simulink library "Px4Library"  (R2015b)
settings: Solver=VariableStepAuto  StartTime=0.0  StopTime=10.0  RelTol=1e-3
undefined symbols (not defined in the file): armed, ctrl_state, INIT_PARAM_VECTOR, mpc_att_sp, mpc_ctrl_state, mpc_manual, mpc_pos_sp_triplet, mpc_vehicle_land_detected, mpc_vehicle_status, v_att_sp, v_control_mode
libraries: simulink x4
(part 2 of 7)

== matlab function Px4Library/mc_att_control/mc_att_control_main ==
  data: hrt_absolute_time input; parameters input; self input Bus: selfBus; selfOut output Bus: selfBus
function selfOut = mc_att_control_main(hrt_absolute_time, parameters, self)
    %#codegen
    % MC_ATT_CONTROL_MAIN Run PX4 attitude controller
    % Based on C++ code retrieved from github.com/px4/Firmware (07/01/17)
    % Created:       07/01/17 by J.X.J. Bannwarth jban039@aucklanduni.ac.nz
    % Last modified: 07/01/17 by J.X.J. Bannwarth jban039@aucklanduni.ac.nz
    %
    % Original disclaimers:
    %
    % %%%%%%%%%%%%%%%%%%%%%%%%%%%%%%%%%%%%%%%%%%%%%%%%%%%%%%%%%%%%%%%%%%%%%%%%%
    %
    %   Copyright (c) 2013-2015 PX4 Development Team. All rights reserved.
    %
    % Redistribution and use in source and binary forms, with or without
    % modification, are permitted provided that the following conditions
    % are met:
    %
    % 1. Redistributions of source code must retain the above copyright
    %    notice, this list of conditions and the following disclaimer.
    % 2. Redistributions in binary form must reproduce the above copyright
    %    notice, this list of conditions and the following disclaimer in
    %    the documentation and/or other materials provided with the
    %    distribution.
    % 3. Neither the name PX4 nor the names of its contributors may be
    %    used to endorse or promote products derived from this software
    %    without specific prior written permission.
    %
    % THIS SOFTWARE IS PROVIDED BY THE COPYRIGHT HOLDERS AND CONTRIBUTORS
    % "AS IS" AND ANY EXPRESS OR IMPLIED WARRANTIES, INCLUDING, BUT NOT
    % LIMITED TO, THE IMPLIED WARRANTIES OF MERCHANTABILITY AND FITNESS
    % FOR A PARTICULAR PURPOSE ARE DISCLAIMED. IN NO EVENT SHALL THE
    % COPYRIGHT OWNER OR CONTRIBUTORS BE LIABLE FOR ANY DIRECT, INDIRECT,
    % INCIDENTAL, SPECIAL, EXEMPLARY, OR CONSEQUENTIAL DAMAGES (INCLUDING,
    % BUT NOT LIMITED TO, PROCUREMENT OF SUBSTITUTE GOODS OR SERVICES; LOSS
    % OF USE, DATA, OR PROFITS; OR BUSINESS INTERRUPTION) HOWEVER CAUSED
    % AND ON ANY THEORY OF LIABILITY, WHETHER IN CONTRACT, STRICT
    % LIABILITY, OR TORT (INCLUDING NEGLIGENCE OR OTHERWISE) ARISING IN
    % ANY WAY OUT OF THE USE OF THIS SOFTWARE, EVEN IF ADVISED OF THE
    % POSSIBILITY OF SUCH DAMAGE.
    %
    % %%%%%%%%%%%%%%%%%%%%%%%%%%%%%%%%%%%%%%%%%%%%%%%%%%%%%%%%%%%%%%%%%%%%%%%%%
    %
    % @file mc_att_control_main.cpp
    % Multicopter attitude controller.
    %
    % Publication for the desired attitude tracking:
    % Daniel Mellinger and Vijay Kumar. Minimum Snap Trajectory Generation and 
    % Control for Quadrotors.
    % Int. Conf. on Robotics and Automation, Shanghai, China, May 2011.
    %
    % @author Lorenz Meier        <lorenz@px4.io>
    % @author Anton Babushkin    <anton.babushkin@me.com>
    % @author Sander Smeets    <sander@droneslab.com>
    %
    % The controller has two loops: P loop for angular error and PD loop for 
    % angular rate error.
    % Desired rotation calculated keeping in mind that yaw response is normally
    % slower than roll/pitch.
    % For small deviations controller rotates copter to have shortest path of
    % thrust vector and independently rotates around yaw,
    % so actual rotation axis is not constant. For large deviations controller
    % rotates copter around fixed axis.
    % These two approaches fused seamlessly with weight depending on angular
    % error.
    % When thrust vector directed near-horizontally (e.g. roll ~= PI/2) yaw
    % setpoint ignored because of singularity.
    % Controller doesn't use Euler angles for work, they generated only for
    % more human-friendly control and logging.
    % If rotation matrix setpoint is invalid it will be generated from Euler
    % angles for compatibility with old position controllers.

    % Multicopter attitude control app start / stop handling function
    %
    % @ingroup apps

    const.YAW_DEADZONE                    = 0.05;
    const.MIN_TAKEOFF_THRUST              = 0.2;
    const.TPA_RATE_LOWER_LIMIT            = 0.05;
    const.MANUAL_THROTTLE_MAX_MULTICOPTER = 0.9;
    const.ATTITUDE_TC_DEFAULT             = 0.2;

    const.AXIS_INDEX_ROLL  = 1;
    const.AXIS_INDEX_PITCH = 2;
    const.AXIS_INDEX_YAW   = 3;
    const.AXIS_COUNT       = 3;

    selfOut = task_main(hrt_absolute_time, parameters, self, const);
end
% class MulticopterAttitudeControl
% {
% public:
%     % /**
%      * Constructor
%      */
%     MulticopterAttitudeControl();
% 
%     % /**
%      * Destructor, also kills the main task
%      */
%     ~MulticopterAttitudeControl();
% 
%     % /**
%      * Start the multicopter attitude control task.
%      *
%      * @return        OK on success.
%      */
%     int        start();
% 
% private:
% 
%     bool    _task_should_exit;        % /**< if true, task_main() should exit */
%     int        _control_task;            % /**< task handle */
% 
%     int        _ctrl_state_sub;        % /**< control state subscription */
%     int        _v_att_sp_sub;            % /**< vehicle attitude setpoint subscription */
%     int        _v_rates_sp_sub;        % /**< vehicle rates setpoint subscription */
%     int        _v_control_mode_sub;    % /**< vehicle control mode subscription */
%     int        _params_sub;            % /**< parameter updates subscription */
%     int        _manual_control_sp_sub;    % /**< manual control setpoint subscription */
%     int        _armed_sub;                % /**< arming status subscription */
%     int        _vehicle_status_sub;    % /**< vehicle status subscription */
%     int     _motor_limits_sub;        % /**< motor limits subscription */
%     int     _battery_status_sub;    % /**< battery status subscription */
% 
%     orb_advert_t    _v_rates_sp_pub;        % /**< rate setpoint publication */
%     orb_advert_t    _actuators_0_pub;        % /**< attitude actuator controls publication */
%     orb_advert_t    _controller_status_pub;    % /**< controller status publication */
% 
%     orb_id_t _rates_sp_id;    % /**< pointer to correct rates setpoint uORB metadata structure */
%     orb_id_t _actuators_id;    % /**< pointer to correct actuator controls0 uORB metadata structure */
% 
%     bool        _actuators_0_circuit_breaker_enabled;    % /**< circuit breaker to suppress output */
% 
%     struct control_state_s                _ctrl_state;        % /**< control state */
%     struct vehicle_attitude_setpoint_s    _v_att_sp;            % /**< vehicle attitude setpoint */
%     struct vehicle_rates_setpoint_s        _v_rates_sp;        % /**< vehicle rates setpoint */
%     struct manual_control_setpoint_s    _manual_control_sp;    % /**< manual control setpoint */
%     struct vehicle_control_mode_s        _v_control_mode;    % /**< vehicle control mode */
%     struct actuator_controls_s            _actuators;            % /**< actuator controls */
%     struct actuator_armed_s                _armed;                % /**< actuator arming status */
%     struct vehicle_status_s                _vehicle_status;    % /**< vehicle status */
%     struct multirotor_motor_limits_s    _motor_limits;        % /**< motor limits */
%     struct mc_att_ctrl_status_s         _controller_status; % /**< controller status */
%     struct battery_status_s                _battery_status;    % /**< battery status */
% 
%     union {
%         struct {
%             uint16_t motor_pos    : 1; % 0 - true when any motor has saturated in the positive direction
%             uint16_t motor_neg    : 1; % 1 - true when any motor has saturated in the negative direction
%             uint16_t roll_pos    : 1; % 2 - true when a positive roll demand change will increase saturation
%             uint16_t roll_neg    : 1; % 3 - true when a negative roll demand change will increase saturation
%             uint16_t pitch_pos    : 1; % 4 - true when a positive pitch demand change will increase saturation
%             uint16_t pitch_neg    : 1; % 5 - true when a negative pitch demand change will increase saturation
%             uint16_t yaw_pos    : 1; % 6 - true when a positive yaw demand change will increase saturation
%             uint16_t yaw_neg    : 1; % 7 - true when a negative yaw demand change will increase saturation
%             uint16_t thrust_pos    : 1; % 8 - true when a positive thrust demand change will increase saturation
%             uint16_t thrust_neg    : 1; % 9 - true when a negative thrust demand change will increase saturation
%         } flags;
%         uint16_t value;
%     } _saturation_status;
% 
%     perf_counter_t    _loop_perf;            % /**< loop performance counter */
%     perf_counter_t    _controller_latency_perf;
% 
%     math::Vector<3>        _rates_prev;    % /**< angular rates on previous step */
%     math::Vector<3>        _rates_sp_prev; % /**< previous rates setpoint */
%     math::Vector<3>        _rates_sp;        % /**< angular rates setpoint */
%     math::Vector<3>        _rates_int;        % /**< angular rates integral error */
%     float                _thrust_sp;        % /**< thrust setpoint */
%     math::Vector<3>        _att_control;    % /**< attitude control vector */
% 
%     math::Matrix<3, 3>  _I;                % /**< identity matrix */
% 
%     struct {
%         param_t roll_p;
%         param_t roll_rate_p;
%         param_t roll_rate_i;
%         param_t roll_rate_integ_lim;
%         param_t roll_rate_d;
%         param_t roll_rate_ff;
%         param_t pitch_p;
%         param_t pitch_rate_p;
%         param_t pitch_rate_i;
%         param_t pitch_rate_integ_lim;
%         param_t pitch_rate_d;
%         param_t pitch_rate_ff;
%         param_t tpa_breakpoint_p;
%         param_t tpa_breakpoint_i;
%         param_t tpa_breakpoint_d;
%         param_t tpa_rate_p;
%         param_t tpa_rate_i;
%         param_t tpa_rate_d;
%         param_t yaw_p;
%         param_t yaw_rate_p;
%         param_t yaw_rate_i;
%         param_t yaw_rate_integ_lim;
%         param_t yaw_rate_d;
%         param_t yaw_rate_ff;
%         param_t yaw_ff;
%         param_t roll_rate_max;
%         param_t pitch_rate_max;
%         param_t yaw_rate_max;
%         param_t yaw_auto_max;
% 
%         param_t acro_roll_max;
%         param_t acro_pitch_max;
%         param_t acro_yaw_max;
%         param_t rattitude_thres;
% 
%         param_t vtol_type;
%         param_t roll_tc;
%         param_t pitch_tc;
%         param_t vtol_opt_recovery_enabled;
%         param_t vtol_wv_yaw_rate_scale;
% 
%         param_t bat_scale_en;
% 
%     }        _params_handles;        % /**< handles for interesting parameters */
% 
%     struct {
%         math::Vector<3> att_p;                    % /**< P gain for angular error */
%         math::Vector<3> rate_p;                % /**< P gain for angular rate error */
%         math::Vector<3> rate_i;                % /**< I gain for angular rate error */
%         math::Vector<3> rate_int_lim;            % /**< integrator state limit for rate loop */
%         math::Vector<3> rate_d;                % /**< D gain for angular rate error */
%         math::Vector<3>    rate_ff;            % /**< Feedforward gain for desired rates */
%         float yaw_ff;                        % /**< yaw control feed-forward */
% 
%         float tpa_breakpoint_p;                % /**< Throttle PID Attenuation breakpoint */
%         float tpa_breakpoint_i;                % /**< Throttle PID Attenuation breakpoint */
%         float tpa_breakpoint_d;                % /**< Throttle PID Attenuation breakpoint */
%         float tpa_rate_p;                    % /**< Throttle PID Attenuation slope */
%         float tpa_rate_i;                    % /**< Throttle PID Attenuation slope */
%         float tpa_rate_d;                    % /**< Throttle PID Attenuation slope */
% 
%         float roll_rate_max;
%         float pitch_rate_max;
%         float yaw_rate_max;
%         float yaw_auto_max;
%         math::Vector<3> mc_rate_max;        % /**< attitude rate limits in stabilized modes */
%         math::Vector<3> auto_rate_max;        % /**< attitude rate limits in auto modes */
%         math::Vector<3> acro_rate_max;        % /**< max attitude rates in acro mode */
%         float rattitude_thres;
%         int vtol_type;                        % /**< 0 = Tailsitter, 1 = Tiltrotor, 2 = Standard airframe */
%         bool vtol_opt_recovery_enabled;
%         float vtol_wv_yaw_rate_scale;            % /**< Scale value [0, 1] for yaw rate setpoint  */
% 
%         int bat_scale_en;
%     }        _params;
% 
%     TailsitterRecovery *_ts_opt_recovery;    % /**< Computes optimal rates for tailsitter recovery */
% 
%     % /**
%      * Update our local parameter cache.
%      */
%     int            parameters_update();
% 
%     % /**
%      * Check for parameter update and handle it.
%      */
%     void        parameter_update_poll();
% 
%     % /**
%      * Check for changes in vehicle control mode.
%      */
%     void        vehicle_control_mode_poll();
% 
%     % /**
%      * Check for changes in manual inputs.
%      */
%     void        vehicle_manual_poll();
% 
%     % /**
%      * Check for attitude setpoint updates.
%      */
%     void        vehicle_attitude_setpoint_poll();
% 
%     % /**
%      * Check for rates setpoint updates.
%      */
%     void        vehicle_rates_setpoint_poll();
% 
%     % /**
%      * Check for arming status updates.
%      */
%     void        arming_status_poll();
% 
%     % /**
%      * Attitude controller.
%      */
%     void        control_attitude(float dt);
% 
%     % /**
%      * Attitude rates controller.
%      */
%     void        control_attitude_rates(float dt);
% 
%     % /**
%      * Throttle PID attenuation.
%      */
%     math::Vector<3> pid_attenuations(float tpa_breakpoint, float tpa_rate);
% 
%     % /**
%      * Check for vehicle status updates.
%      */
%     void        vehicle_status_poll();
% 
%     % /**
%      * Check for vehicle motor limits status.
%      */
%     void        vehicle_motor_limits_poll();
% 
%     % /**
%      * Check for battery status updates.
%      */
%     void        battery_status_poll();
% 
%     % /**
%      * Shim for calling task_main from task_create.
%      */
%     static void    task_main_trampoline(int argc, char *argv[]);
% 
%     % /**
%      * Main attitude control task.
%      */
%     void        task_main();
% };
% 
% namespace mc_att_control
% {
% 
% MulticopterAttitudeControl    *g_control;
% }
% 
% MulticopterAttitudeControl::MulticopterAttitudeControl() :
% 
%     _task_should_exit(false),
%     _control_task(-1),
% 
%     % /* subscriptions */
%     _ctrl_state_sub(-1),
%     _v_att_sp_sub(-1),
%     _v_control_mode_sub(-1),
%     _params_sub(-1),
%     _manual_control_sp_sub(-1),
%     _armed_sub(-1),
%     _vehicle_status_sub(-1),
% 
%     % /* publications */
%     _v_rates_sp_pub(nullptr),
%     _actuators_0_pub(nullptr),
%     _controller_status_pub(nullptr),
%     _rates_sp_id(0),
%     _actuators_id(0),
% 
%     _actuators_0_circuit_breaker_enabled(false),
% 
%     _ctrl_state{},
%     _v_att_sp{},
%     _v_rates_sp{},
%     _manual_control_sp{},
%     _v_control_mode{},
%     _actuators{},
%     _armed{},
%     _vehicle_status{},
%     _motor_limits{},
%     _controller_status{},
%     _battery_status{},
% 
%     _saturation_status{},
%     % /* performance counters */
%     _loop_perf(perf_alloc(PC_ELAPSED, "mc_att_control")),
%     _controller_latency_perf(perf_alloc_once(PC_ELAPSED, "ctrl_latency")),
%     _ts_opt_recovery(nullptr)
% 
% {
%     _vehicle_status.is_rotary_wing = true;
% 
%     _params.att_p.zero();
%     _params.rate_p.zero();
%     _params.rate_i.zero();
%     _params.rate_int_lim.zero();
%     _params.rate_d.zero();
%     _params.rate_ff.zero();
%     _params.yaw_ff = 0.0f;
%     _params.roll_rate_max = 0.0f;
%     _params.pitch_rate_max = 0.0f;
%     _params.yaw_rate_max = 0.0f;
%     _params.mc_rate_max.zero();
%     _params.auto_rate_max.zero();
%     _params.acro_rate_max.zero();
%     _params.rattitude_thres = 1.0f;
%     _params.vtol_opt_recovery_enabled = false;
%     _params.vtol_wv_yaw_rate_scale = 1.0f;
%     _params.bat_scale_en = 0;
% 
%     _rates_prev.zero();
%     _rates_sp.zero();
%     _rates_sp_prev.zero();
%     _rates_int.zero();
%     _thrust_sp = 0.0f;
%     _att_control.zero();
% 
%     _I.identity();
% 
%     _params_handles.roll_p                    = param_find("MC_ROLL_P");
%     _params_handles.roll_rate_p               = param_find("MC_ROLLRATE_P");
%     _params_handles.roll_rate_i               = param_find("MC_ROLLRATE_I");
%     _params_handles.roll_rate_integ_lim       = param_find("MC_RR_INT_LIM");
%     _params_handles.roll_rate_d               = param_find("MC_ROLLRATE_D");
%     _params_handles.roll_rate_ff              = param_find("MC_ROLLRATE_FF");
%     _params_handles.pitch_p                   = param_find("MC_PITCH_P");
%     _params_handles.pitch_rate_p              = param_find("MC_PITCHRATE_P");
%     _params_handles.pitch_rate_i              = param_find("MC_PITCHRATE_I");
%     _params_handles.pitch_rate_integ_lim      = param_find("MC_PR_INT_LIM");
%     _params_handles.pitch_rate_d              = param_find("MC_PITCHRATE_D");
%     _params_handles.pitch_rate_ff             = param_find("MC_PITCHRATE_FF");
%     _params_handles.tpa_breakpoint_p          = param_find("MC_TPA_BREAK_P");
%     _params_handles.tpa_breakpoint_i          = param_find("MC_TPA_BREAK_I");
%     _params_handles.tpa_breakpoint_d          = param_find("MC_TPA_BREAK_D");
%     _params_handles.tpa_rate_p                = param_find("MC_TPA_RATE_P");
%     _params_handles.tpa_rate_i                = param_find("MC_TPA_RATE_I");
%     _params_handles.tpa_rate_d                = param_find("MC_TPA_RATE_D");
%     _params_handles.yaw_p                     = param_find("MC_YAW_P");
%     _params_handles.yaw_rate_p                = param_find("MC_YAWRATE_P");
%     _params_handles.yaw_rate_i                = param_find("MC_YAWRATE_I");
%     _params_handles.yaw_rate_integ_lim        = param_find("MC_YR_INT_LIM");
%     _params_handles.yaw_rate_d                = param_find("MC_YAWRATE_D");
%     _params_handles.yaw_rate_ff               = param_find("MC_YAWRATE_FF");
%     _params_handles.yaw_ff                    = param_find("MC_YAW_FF");
%     _params_handles.roll_rate_max             = param_find("MC_ROLLRATE_MAX");
%     _params_handles.pitch_rate_max            = param_find("MC_PITCHRATE_MAX");
%     _params_handles.yaw_rate_max              = param_find("MC_YAWRATE_MAX");
%     _params_handles.yaw_auto_max              = param_find("MC_YAWRAUTO_MAX");
%     _params_handles.acro_roll_max             = param_find("MC_ACRO_R_MAX");
%     _params_handles.acro_pitch_max            = param_find("MC_ACRO_P_MAX");
%     _params_handles.acro_yaw_max              = param_find("MC_ACRO_Y_MAX");
%     _params_handles.rattitude_thres           = param_find("MC_RATT_TH");
%     _params_handles.vtol_type                 = param_find("VT_TYPE");
%     _params_handles.roll_tc                   = param_find("MC_ROLL_TC");
%     _params_handles.pitch_tc                  = param_find("MC_PITCH_TC");
%     _params_handles.vtol_opt_recovery_enabled = param_find("VT_OPT_RECOV_EN");
%     _params_handles.vtol_wv_yaw_rate_scale    = param_find("VT_WV_YAWR_SCL");
%     _params_handles.bat_scale_en              = param_find("MC_BAT_SCALE_EN");
% 
% 
% 
%     % /* fetch initial parameter values */
%     parameters_update();
% 
%     if (_params.vtol_type == 0 && _params.vtol_opt_recovery_enabled) {
%         % the vehicle is a tailsitter, use optimal recovery control strategy
%         _ts_opt_recovery = new TailsitterRecovery();
%     }
% 
% 
% }
% 

% MulticopterAttitudeControl::~MulticopterAttitudeControl()
% {
%     if (_control_task != -1) {
%         % /* task wakes up every 100ms or so at the longest */
%         _task_should_exit = true;
% 
%         % /* wait for a second for the task to quit at our request */
%         unsigned i = 0;
% 
%         do {
%             % /* wait 20ms */
%             usleep(20000);
% 
%             % /* if we have given up, kill it */
%             if (++i > 50) {
%                 px4_task_delete(_control_task);
%                 break;
%             }
%         } while (_control_task != -1);
%     }
% 
%     if (_ts_opt_recovery != nullptr) {
%         delete _ts_opt_recovery;
%     }
% 
%     mc_att_control::g_control = nullptr;
% }
% 
% int
% MulticopterAttitudeControl::

%% Parameters_update
function self = parameters_update( parameters, self, const )
    
    roll_tc         = parameters.MC_ROLL_TC;
    pitch_tc        = parameters.MC_PITCH_TC; 
    roll_p          = parameters.MC_ROLL_P;
    roll_rate_p     = parameters.MC_ROLLRATE_P;
    roll_rate_i     = parameters.MC_ROLLRATE_I;
    roll_rate_d     = parameters.MC_ROLLRATE_D;
    roll_rate_ff    = parameters.MC_ROLLRATE_FF;
    pitch_p         = parameters.MC_PITCH_P;
    pitch_rate_p    = parameters.MC_PITCHRATE_P;
    pitch_rate_i    = parameters.MC_PITCHRATE_I;
    pitch_rate_d    = parameters.MC_PITCHRATE_D;
    pitch_rate_ff   = parameters.MC_PITCHRATE_FF;
    yaw_p           = parameters.MC_YAW_P;
    yaw_rate_p      = parameters.MC_YAWRATE_P;
    yaw_rate_i      = parameters.MC_YAWRATE_I;
    yaw_rate_d      = parameters.MC_YAWRATE_D;
    yaw_rate_ff     = parameters.MC_YAWRATE_FF;
    roll_rate_max   = parameters.MC_ROLLRATE_MAX;
    pitch_rate_max  = parameters.MC_PITCHRATE_MAX;
    yaw_rate_max    = parameters.MC_YAWRATE_MAX;
    yaw_auto_max    = parameters.MC_YAWRAUTO_MAX;
    acro_roll_max   = parameters.MC_ACRO_R_MAX;
    acro_pitch_max  = parameters.MC_ACRO_P_MAX;
    acro_yaw_max    = parameters.MC_ACRO_Y_MAX;

    % Roll gains
    self.params.att_p(1)        = roll_p * (const.ATTITUDE_TC_DEFAULT / roll_tc);
    self.params.rate_p(1)       = roll_rate_p * (const.ATTITUDE_TC_DEFAULT / roll_tc);
    self.params.rate_i(1)       = roll_rate_i;
    self.params.rate_int_lim(1) = parameters.MC_RR_INT_LIM;
    self.params.rate_d(1)       = roll_rate_d * (const.ATTITUDE_TC_DEFAULT / roll_tc);
    self.params.rate_ff(1)      = roll_rate_ff;
    
    % Pitch gains
    self.params.att_p(2)        = pitch_p * (const.ATTITUDE_TC_DEFAULT / pitch_tc);
    self.params.rate_p(2)       = pitch_rate_p * (const.ATTITUDE_TC_DEFAULT / pitch_tc);
    self.params.rate_i(2)       = pitch_rate_i;
    self.params.rate_int_lim(2) = parameters.MC_PR_INT_LIM;
    self.params.rate_d(2)       = pitch_rate_d * (const.ATTITUDE_TC_DEFAULT / pitch_tc);
    self.params.rate_ff(2)      = pitch_rate_ff;

    self.params.tpa_breakpoint_p = parameters.MC_TPA_BREAK_P;
    self.params.tpa_breakpoint_i = parameters.MC_TPA_BREAK_I;
    self.params.tpa_breakpoint_d = parameters.MC_TPA_BREAK_D;

    self.params.tpa_rate_p = parameters.MC_TPA_RATE_P;
    self.params.tpa_rate_i = parameters.MC_TPA_RATE_I;
    self.params.tpa_rate_d = parameters.MC_TPA_RATE_D;
    
    % Yaw gains
    self.params.att_p(3)        = yaw_p;
    self.params.rate_p(3)       = yaw_rate_p;
    self.params.rate_i(3)       = yaw_rate_i;
    self.params.rate_int_lim(3) = parameters.MC_YR_INT_LIM;
    self.params.rate_d(3)       = yaw_rate_d;
    self.params.rate_ff(3)      = yaw_rate_ff;
    
    self.params.yaw_ff          = parameters.MC_YAW_FF;
    
    % Angular rate limits
    self.params.mc_rate_max(1) = radians( roll_rate_max );
    self.params.mc_rate_max(2) = radians( pitch_rate_max );
    self.params.mc_rate_max(3) = radians( yaw_rate_max );

    % Auto angular rate limits
    self.params.auto_rate_max(1) = radians( roll_rate_max );
    self.params.auto_rate_max(2) = radians( pitch_rate_max );
    self.params.auto_rate_max(3) = radians( yaw_auto_max );

    % Manual rate control scale and auto mode roll/pitch rate limits
    self.params.acro_rate_max(1) = radians( acro_roll_max );
    self.params.acro_rate_max(2) = radians( acro_pitch_max );
    self.params.acro_rate_max(3) = radians( acro_yaw_max );

    % Stick deflection needed in rattitude mode to control rates not angles
    self.params.rattitude_thres = parameters.MC_RATT_TH;

    self.params.vtol_type                 = parameters.VT_TYPE;
    self.params.vtol_wv_yaw_rate_scale    = parameters.VT_WV_YAWR_SCL;
    self.params.vtol_opt_recovery_enabled = parameters.VT_OPT_RECOV_EN;

    self.params.bat_scale_en = parameters.MC_BAT_SCALE_EN;
    
    self.params.actuators_0_circuit_breaker_enabled = 0;
end

% {
%     float v;
% 
%     float roll_tc, pitch_tc;
% 
%     param_get(_params_handles.roll_tc, &roll_tc);
%     param_get(_params_handles.pitch_tc, &pitch_tc);
% 
%     % /* roll gains */
%     param_get(_params_handles.roll_p, &v);
%     _params.att_p(0) = v * (ATTITUDE_TC_DEFAULT / roll_tc);
%     param_get(_params_handles.roll_rate_p, &v);
%     _params.rate_p(0) = v * (ATTITUDE_TC_DEFAULT / roll_tc);
%     param_get(_params_handles.roll_rate_i, &v);
%     _params.rate_i(0) = v;
%     param_get(_params_handles.roll_rate_integ_lim, &v);
%     _params.rate_int_lim(0) = v;
%     param_get(_params_handles.roll_rate_d, &v);
%     _params.rate_d(0) = v * (ATTITUDE_TC_DEFAULT / roll_tc);
%     param_get(_params_handles.roll_rate_ff, &v);
%     _params.rate_ff(0) = v;
% 
%     % /* pitch gains */
%     param_get(_params_handles.pitch_p, &v);
%     _params.att_p(1) = v * (ATTITUDE_TC_DEFAULT / pitch_tc);
%     param_get(_params_handles.pitch_rate_p, &v);
%     _params.rate_p(1) = v * (ATTITUDE_TC_DEFAULT / pitch_tc);
%     param_get(_params_handles.pitch_rate_i, &v);
%     _params.rate_i(1) = v;
%     param_get(_params_handles.pitch_rate_integ_lim, &v);
%     _params.rate_int_lim(1) = v;
%     param_get(_params_handles.pitch_rate_d, &v);
%     _params.rate_d(1) = v * (ATTITUDE_TC_DEFAULT / pitch_tc);
%     param_get(_params_handles.pitch_rate_ff, &v);
%     _params.rate_ff(1) = v;
% 
%     param_get(_params_handles.tpa_breakpoint_p, &_params.tpa_breakpoint_p);
%     param_get(_params_handles.tpa_breakpoint_i, &_params.tpa_breakpoint_i);
%     param_get(_params_handles.tpa_breakpoint_d, &_params.tpa_breakpoint_d);
%     param_get(_params_handles.tpa_rate_p, &_params.tpa_rate_p);
%     param_get(_params_handles.tpa_rate_i, &_params.tpa_rate_i);
%     param_get(_params_handles.tpa_rate_d, &_params.tpa_rate_d);
% 
%     % /* yaw gains */
%     param_get(_params_handles.yaw_p, &v);
%     _params.att_p(2) = v;
%     param_get(_params_handles.yaw_rate_p, &v);
%     _params.rate_p(2) = v;
%     param_get(_params_handles.yaw_rate_i, &v);
%     _params.rate_i(2) = v;
%     param_get(_params_handles.yaw_rate_integ_lim, &v);
%     _params.rate_int_lim(2) = v;
%     param_get(_params_handles.yaw_rate_d, &v);
%     _params.rate_d(2) = v;
%     param_get(_params_handles.yaw_rate_ff, &v);
%     _params.rate_ff(2) = v;
% 
%     param_get(_params_handles.yaw_ff, &_params.yaw_ff);
% 
%     % /* angular rate limits */
%     param_get(_params_handles.roll_rate_max, &_params.roll_rate_max);
%     _params.mc_rate_max(0) = math::radians(_params.roll_rate_max);
%     param_get(_params_handles.pitch_rate_max, &_params.pitch_rate_max);
%     _params.mc_rate_max(1) = math::radians(_params.pitch_rate_max);
%     param_get(_params_handles.yaw_rate_max, &_params.yaw_rate_max);
%     _params.mc_rate_max(2) = math::radians(_params.yaw_rate_max);
% 
%     % /* auto angular rate limits */
%     param_get(_params_handles.roll_rate_max, &_params.roll_rate_max);
%     _params.auto_rate_max(0) = math::radians(_params.roll_rate_max);
%     param_get(_params_handles.pitch_rate_max, &_params.pitch_rate_max);
%     _params.auto_rate_max(1) = math::radians(_params.pitch_rate_max);
%     param_get(_params_handles.yaw_auto_max, &_params.yaw_auto_max);
%     _params.auto_rate_max(2) = math::radians(_params.yaw_auto_max);
% 
%     % /* manual rate control scale and auto mode roll/pitch rate limits */
%     param_get(_params_handles.acro_roll_max, &v);
%     _params.acro_rate_max(0) = math::radians(v);
%     param_get(_params_handles.acro_pitch_max, &v);
%     _params.acro_rate_max(1) = math::radians(v);
%     param_get(_params_handles.acro_yaw_max, &v);
%     _params.acro_rate_max(2) = math::radians(v);
% 
%     % /* stick deflection needed in rattitude mode to control rates not angles */
%     param_get(_params_handles.rattitude_thres, &_params.rattitude_thres);
% 
%     param_get(_params_handles.vtol_type, &_params.vtol_type);
% 
%     int tmp;
%     param_get(_params_handles.vtol_opt_recovery_enabled, &tmp);
%     _params.vtol_opt_recovery_enabled = (bool)tmp;
% 
%     param_get(_params_handles.vtol_wv_yaw_rate_scale, &_params.vtol_wv_yaw_rate_scale);
% 
%     param_get(_params_handles.bat_scale_en, &_params.bat_scale_en);
% 
%     _actuators_0_circuit_breaker_enabled = circuit_breaker_enabled("CBRK_RATE_CTRL", CBRK_RATE_CTRL_KEY);
% 
%     return OK;
% }
% 
% void
% MulticopterAttitudeControl::parameter_update_poll()
% {
%     bool updated;
% 
%     % /* Check if parameters have changed */
%     orb_check(_params_sub, &updated);
% 
%     if (updated) {
%         struct parameter_update_s param_update;
%         orb_copy(ORB_ID(parameter_update), _params_sub, &param_update);
%         parameters_update();
%     }
% }
% 
% void
% MulticopterAttitudeControl::vehicle_control_mode_poll()
% {
%     bool updated;
% 
%     % /* Check if vehicle control mode has changed */
%     orb_check(_v_control_mode_sub, &updated);
% 
%     if (updated) {
%         orb_copy(ORB_ID(vehicle_control_mode), _v_control_mode_sub, &_v_control_mode);
%     }
% }
% 
% void
% MulticopterAttitudeControl::vehicle_manual_poll()
% {
%     bool updated;
% 
%     % /* get pilots inputs */
%     orb_check(_manual_control_sp_sub, &updated);
% 
%     if (updated) {
%         orb_copy(ORB_ID(manual_control_setpoint), _manual_control_sp_sub, &_manual_control_sp);
%     }
% }
% 
% void
% MulticopterAttitudeControl::vehicle_attitude_setpoint_poll()
% {
%     % /* check if there is a new setpoint */
%     bool updated;
%     orb_check(_v_att_sp_sub, &updated);
% 
%     if (updated) {
%         orb_copy(ORB_ID(vehicle_attitude_setpoint), _v_att_sp_sub, &_v_att_sp);
%     }
% }
% 
% void
% MulticopterAttitudeControl::vehicle_rates_setpoint_poll()
% {
%     % /* check if there is a new setpoint */
%     bool updated;
%     orb_check(_v_rates_sp_sub, &updated);
% 
%     if (updated) {
%         orb_copy(ORB_ID(vehicle_rates_setpoint), _v_rates_sp_sub, &_v_rates_sp);
%     }
% }
% 
% void
% MulticopterAttitudeControl::arming_status_poll()
% {
%     % /* check if there is a new setpoint */
%     bool updated;
%     orb_check(_armed_sub, &updated);
% 
%     if (updated) {
%         orb_copy(ORB_ID(actuator_armed), _armed_sub, &_armed);
%     }
% }
% 
% void
% MulticopterAttitudeControl::vehicle_status_poll()
% {
%     % /* check if there is new status information */
%     bool vehicle_status_updated;
%     orb_check(_vehicle_status_sub, &vehicle_status_updated);
% 
%     if (vehicle_status_updated) {
%         orb_copy(ORB_ID(vehicle_status), _vehicle_status_sub, &_vehicle_status);
% 
%         % /* set correct uORB ID, depending on if vehicle is VTOL or not */
%         if (!_rates_sp_id) {
%             if (_vehicle_status.is_vtol) {
%                 _rates_sp_id = ORB_ID(mc_virtual_rates_setpoint);
%                 _actuators_id = ORB_ID(actuator_controls_virtual_mc);
% 
%             } else {
%                 _rates_sp_id = ORB_ID(vehicle_rates_setpoint);
%                 _actuators_id = ORB_ID(actuator_controls_0);
%             }
%         }
%     }
% }
% 
% void
% MulticopterAttitudeControl::vehicle_motor_limits_poll()
% {
%     % /* check if there is a new message */
%     bool updated;
%     orb_check(_motor_limits_sub, &updated);
% 
%     if (updated) {
%         orb_copy(ORB_ID(multirotor_motor_limits), _motor_limits_sub, &_motor_limits);
%         _saturation_status.value = _motor_limits.saturation_status;
%     }
% }
% 
% void
% MulticopterAttitudeControl::battery_status_poll()
% {
%     % /* check if there is a new message */
%     bool updated;
%     orb_check(_battery_status_sub, &updated);
% 
%     if (updated) {
%         orb_copy(ORB_ID(battery_status), _battery_status_sub, &_battery_status);
%     }
% }

%% Attitude controller.
% void
function self = control_attitude(self)
% CONTROL_ATTITUDE Calculate attitude rate setpoints
%  * Input: 'vehicle_attitude_setpoint' topics (depending on mode)
%  * Output: '_rates_sp' vector, '_thrust_sp'

    % vehicle_attitude_setpoint_poll();

    self.thrust_sp = self.v_att_sp.thrust;

    % /* construct attitude setpoint rotation matrix */
    q_sp = [ self.v_att_sp.q_d(1); ...
             self.v_att_sp.q_d(2); ...
             self.v_att_sp.q_d(3); ...
             self.v_att_sp.q_d(4)]; % math::Quaternion
    R_sp = to_dcm( q_sp ); % math::Matrix<3, 3>

    % /* get current rotation matrix from control state quaternions */
    q_att = [self.ctrl_state.q(1); ...
             self.ctrl_state.q(2); ...
             self.ctrl_state.q(3); ...
             self.ctrl_state.q(4)]; % math::Quaternion
    R = to_dcm( q_att ); % math::Matrix<3, 3>

    % /* all input data is ready, run controller itself */

    % /* try to move thrust vector shortest way, because yaw response is slower than roll/pitch */
    R_z    = [R(1, 3); R(2, 3); R(3, 3)];          % math::Vector<3>
    R_sp_z = [R_sp(1, 3); R_sp(2, 3); R_sp(3, 3)]; % math::Vector<3>

    % /* axis and sin(angle) of desired rotation */
    e_R = R' * cross(R_z, R_sp_z); % math::Vector<3> R.transposed() -> R'

    % /* calculate angle error */
    e_R_z_sin = norm(e_R); % float
    e_R_z_cos = dot(R_z, R_sp_z); % float

    % /* calculate weight for yaw control */
    yaw_w = R_sp(3, 3) * R_sp(3, 3); % float

    % /* calculate rotation matrix after roll/pitch only rotation */
    %R_rp = zeros(3,3); % math::Matrix<3, 3>

    if (e_R_z_sin > 0.0)
        % /* get axis-angle representation */
        e_R_z_angle = atan2(e_R_z_sin, e_R_z_cos); % float
        e_R_z_axis = e_R ./ e_R_z_sin; % math::Vector<3>

        e_R = e_R_z_axis .* e_R_z_angle;

        % /* cross product matrix for e_R_axis */
        % math::Matrix<3, 3> e_R_cp;
        e_R_cp = zeros(3,3);
        e_R_cp(1, 2) = -e_R_z_axis(3);
        e_R_cp(1, 3) =  e_R_z_axis(2);
        e_R_cp(2, 1) =  e_R_z_axis(3);
        e_R_cp(2, 3) = -e_R_z_axis(1);
        e_R_cp(3, 1) = -e_R_z_axis(2);
        e_R_cp(3, 2) =  e_R_z_axis(1);

        % /* rotation matrix for roll/pitch only rotation */
        R_rp = R * ( eye(3,3) + e_R_cp * e_R_z_sin + e_R_cp * e_R_cp * (1.0 - e_R_z_cos) ); % _I -> eye(3,3)
    else
        % /* zero roll/pitch rotation */
        R_rp = R;
    end

    % /* R_rp and R_sp has the same Z axis, calculate yaw error */
    R_sp_x = [ R_sp(1, 1); R_sp(2, 1); R_sp(3, 1) ]; % math::Vector<3> 
    R_rp_x = [ R_rp(1, 1); R_rp(2, 1); R_rp(3, 1) ]; % math::Vector<3>
    e_R(3) = atan2( dot( cross(R_rp_x, R_sp_x), R_sp_z), dot(R_rp_x, R_sp_x) ) * yaw_w;

    if ( e_R_z_cos < 0.0 )
        % /* for large thrust vector rotations use another rotation method:
        % * calculate angle and axis for R -> R_sp rotation directly */
        % q_error; math::Quaternion
        q_error = from_dcm( R' * R_sp ); %.transposed() -> '
        
        % e_R_d = q_error(0) >= 0.0 ? q_error.imag()  * 2.0f : -q_error.imag() * 2.0f; % math::Vector<3>
        if ( q_error(1) >= 0.0 )
            e_R_d =  q_error(2:end) * 2.0; % Still not 100% sure
        else
            e_R_d = -q_error(2:end) * 2.0;
        end
        
        
        % /* use fusion of Z axis based rotation and direct rotation */
        direct_w = e_R_z_cos * e_R_z_cos * yaw_w;
        e_R = e_R * (1.0 - direct_w) + e_R_d * direct_w;
    end

    % /* calculate angular rates setpoint */
    self.rates_sp = self.params.att_p .* e_R;

    % /* limit rates */
    for i = 1:3
        if ( (self.v_control_mode.flag_control_velocity_enabled || self.v_control_mode.flag_control_auto_enabled) && ...
             ~self.v_control_mode.flag_control_manual_enabled)
            self.rates_sp(i) = constrain(self.rates_sp(i), -self.params.auto_rate_max(i), self.params.auto_rate_max(i));
        else
            self.rates_sp(i) = constrain(self.rates_sp(i), -self.params.mc_rate_max(i), self.params.mc_rate_max(i));
        end
    end

    % /* feed forward yaw setpoint rate */
    self.rates_sp(3) = self.rates_sp(3) + self.v_att_sp.yaw_sp_move_rate * yaw_w * self.params.yaw_ff;

    % /* weather-vane mode, dampen yaw rate */
    if ( (self.v_control_mode.flag_control_velocity_enabled || self.v_control_mode.flag_control_auto_enabled) && ...
         (self.v_att_sp.disable_mc_yaw_control == true && ~self.v_control_mode.flag_control_manual_enabled) )
    
        wv_yaw_rate_max = self.params.auto_rate_max(3) * self.params.vtol_wv_yaw_rate_scale; % float
        self.rates_sp(3) = constrain(self.rates_sp(3), -wv_yaw_rate_max, wv_yaw_rate_max);
        
        % prevent integrator winding up in weathervane mode
        self.rates_int(3) = 0.0;
    end

end

%% Throttle PID attenuation
% math::Vector<3>
function pidAttenuationPerAxis = pid_attenuations(tpa_breakpoint, tpa_rate, ...
    self, const) % float, float
% PID_ATTENUATIONS Find attenuation factor
%  * Function visualization available here: https://www.desmos.com/calculator/gn4mfoddje
%  * Input: 'tpa_breakpoint', 'tpa_rate', '_thrust_sp'
%  * Output: 'pidAttenuationPerAxis' vector

     % /* throttle pid attenuation factor */
     tpa = 1.0 - tpa_rate * ( abs(self.v_rates_sp.thrust) - tpa_breakpoint) / (1.0 - tpa_breakpoint); % pidAttenuationPerAxis
     tpa = max( const.TPA_RATE_LOWER_LIMIT, min(1.0, tpa) );

     pidAttenuationPerAxis = zeros(3,1); % math::Vector<3>
     pidAttenuationPerAxis(const.AXIS_INDEX_ROLL) = tpa;
     pidAttenuationPerAxis(const.AXIS_INDEX_PITCH) = tpa;
     pidAttenuationPerAxis(const.AXIS_INDEX_YAW) = 1.0;
    
%     return pidAttenuationPerAxis;
end

%% Attitude rates controller.
% void
function self = control_attitude_rates( dt, self, const ) % dt
% CONTROL_ATTITUDE_RATES Calculate normalized commands
%  * Input: '_rates_sp' vector, '_thrust_sp'
%  * Output: '_att_control' vector

    % /* reset integral if disarmed */
    if (~self.armed.armed || ~self.vehicle_status.is_rotary_wing)
        self.rates_int = self.rates_int .* 0;
    end

    % /* current body angular rates */
    rates = zeros(3,1); % math::Vector<3>
    rates(1) = self.ctrl_state.roll_rate;
    rates(2) = self.ctrl_state.pitch_rate;
    rates(3) = self.ctrl_state.yaw_rate;

    rates_p_scaled = self.params.rate_p .* pid_attenuations(self.params.tpa_breakpoint_p, self.params.tpa_rate_p, self, const); % math::Vector<3>
    rates_i_scaled = self.params.rate_i .* pid_attenuations(self.params.tpa_breakpoint_i, self.params.tpa_rate_i, self, const); % math::Vector<3>
    rates_d_scaled = self.params.rate_d .* pid_attenuations(self.params.tpa_breakpoint_d, self.params.tpa_rate_d, self, const); % math::Vector<3>

    % /* angular rates error */
    rates_err = self.rates_sp - rates; % math::Vector<3>

    self.att_control = rates_p_scaled .* rates_err + ...
               self.rates_int + ...
               rates_d_scaled .* (self.rates_prev - rates) ./ dt + ...
               self.params.rate_ff .* self.rates_sp;

    self.rates_sp_prev = self.rates_sp;
    self.rates_prev = rates;

    % /* update integral only if motors are providing enough thrust to be effective */
    if ( self.thrust_sp > const.MIN_TAKEOFF_THRUST )
        for i = const.AXIS_INDEX_ROLL:const.AXIS_COUNT
            % Check for positive control saturation
            positive_saturation = ...
                ((i == const.AXIS_INDEX_ROLL)  && self.saturation_status.flags.roll_pos) || ...
                ((i == const.AXIS_INDEX_PITCH) && self.saturation_status.flags.pitch_pos) || ...
                ((i == const.AXIS_INDEX_YAW)   && self.saturation_status.flags.yaw_pos); % bool

            % Check for negative control saturation
            negative_saturation = ...
                ((i == const.AXIS_INDEX_ROLL)  && self.saturation_status.flags.roll_neg) || ...
                ((i == const.AXIS_INDEX_PITCH) && self.saturation_status.flags.pitch_neg) || ...
                ((i == const.AXIS_INDEX_YAW)   && self.saturation_status.flags.yaw_neg); % bool

            % prevent further positive control saturation
            if (positive_saturation)
                rates_err(i) = min(rates_err(i), 0.0);
            end

            % prevent further negative control saturation
            if (negative_saturation)
                rates_err(i) = max(rates_err(i), 0.0);
            end

            % Perform the integration using a first order method and do not propaate the result if out of range or invalid
            rate_i = self.rates_int(i) + self.params.rate_i(i) * rates_err(i) * dt; % float

            if (~isinf(rate_i) && (rate_i > -self.params.rate_int_lim(i)) && (rate_i < self.params.rate_int_lim(i)) )
                self.rates_int(i) = rate_i;
            end
        end
    end

    % /* explicitly limit the integrator state */
    for i = const.AXIS_INDEX_ROLL:const.AXIS_COUNT
        self.rates_int(i) = constrain(self.rates_int(i), -self.params.rate_int_lim(i), self.params.rate_int_lim(i));
    end
end

% 
% void
% MulticopterAttitudeControl::task_main_trampoline(int argc, char *argv[])
% {
%     mc_att_control::g_control->task_main();
% }
%

%% Main task
% void
function self = task_main(hrt_absolute_time, parameters, self, const)
% TASK_MAIN Run the other elements of the controller
% Original code uses infinte while loop -> change to single-run through
% loop

    % /* initialize parameters cache - just once */
    if (~self.init)
        self = parameters_update(parameters, self, const);
        self.init = 1;
    end
    
    %if ((hrt_absolute_time/1000000) > 0.5)
    %    disp('hay')
    %end
    
    dt = (hrt_absolute_time - self.last_run) / 1000000.0; % hrt_absolute_time() -> hrt_absolute_time
    self.last_run = hrt_absolute_time;

    % /* guard against too small (< 2ms) and too large (> 20ms) dt's */
    if (dt < 0.002)
        dt = 0.002;
    elseif (dt > 0.02)
        dt = 0.02;
    end

    if (self.v_control_mode.flag_control_attitude_enabled)

        % the  tailsitter recovery instance has not been created, thus, the vehicle
        % is not a tailsitter, do normal attitude control
        self = control_attitude(self);

        % /* publish attitude rates setpoint */
        self.v_rates_sp.roll      = self.rates_sp(1);
        self.v_rates_sp.pitch     = self.rates_sp(2);
        self.v_rates_sp.yaw       = self.rates_sp(3);
        self.v_rates_sp.thrust    = self.thrust_sp;
        self.v_rates_sp.timestamp = hrt_absolute_time;

    else
        % /* attitude controller disabled, poll rates setpoint topic */
        if (self.v_control_mode.flag_control_manual_enabled)
            % /* manual rates control - ACRO mode */
            self.rates_sp = [ self.manual_control_sp.y;
                             -self.manual_control_sp.x;
                              self.manual_control_sp.r] .* self.params.acro_rate_max; % math::Vector<3>
                       
            self.thrust_sp = min(self.manual_control_sp.z, const.MANUAL_THROTTLE_MAX_MULTICOPTER);

            % /* publish attitude rates setpoint */
            self.v_rates_sp.roll      = self.rates_sp(1);
            self.v_rates_sp.pitch     = self.rates_sp(2);
            self.v_rates_sp.yaw       = self.rates_sp(3);
            self.v_rates_sp.thrust    = self.thrust_sp;
            self.v_rates_sp.timestamp = hrt_absolute_time;
        else
            % /* attitude controller disabled, poll rates setpoint topic */
            self.rates_sp(1) = self.v_rates_sp.roll;
            self.rates_sp(2) = self.v_rates_sp.pitch;
            self.rates_sp(3) = self.v_rates_sp.yaw;
            self.thrust_sp   = self.v_rates_sp.thrust;
        end
    end

    if (self.v_control_mode.flag_control_rates_enabled)
        
        self = control_attitude_rates(dt, self, const);

        % /* publish actuator controls */
        self.actuators.control(1) = zero_if_inf( self.att_control(1) );
        self.actuators.control(2) = zero_if_inf( self.att_control(2) );
        self.actuators.control(3) = zero_if_inf( self.att_control(3) );
        self.actuators.control(4) = zero_if_inf( self.thrust_sp );
        self.actuators.control(8) = self.v_att_sp.landing_gear;

        self.actuators.timestamp = hrt_absolute_time;
        self.actuators.timestamp_sample = self.ctrl_state.timestamp;

        % /* scale effort by battery status */
        if (self.params.bat_scale_en && (self.battery_status.scale > 0.0) )
            for i = 1:4
                self.actuators.control(i) = self.actuators.control(i) * self.battery_status.scale;
            end
        end

        self.controller_status.roll_rate_integ  = self.rates_int(1);
        self.controller_status.pitch_rate_integ = self.rates_int(2);
        self.controller_status.yaw_rate_integ   = self.rates_int(3);
        self.controller_status.timestamp        = hrt_absolute_time;
    end
end

%% Other useful functions
function rad = radians( deg )
    rad = deg .* pi ./ 180;
end

function y = constrain( x, x_min, x_max )
    y = max( min(x, x_max), x_min );
end

function out = zero_if_inf(in)
    if ( isinf(in) || isnan(in) )
        out = 0;
    else
        out = in;
    end
end

function R  = to_dcm( data )
    % TO_DCM Convert quaternion to DCM
    % From https://github.com/PX4/Firmware/blob/master/src/lib/mathlib/math/Quaternion.hpp
    aSq = data(1) * data(1);
    bSq = data(2) * data(2);
    cSq = data(3) * data(3);
    dSq = data(4) * data(4);
    R = zeros(3,3);
    R(1,1) = aSq + bSq - cSq - dSq;
    R(1,2) = 2.0 * ( data(2) * data(3) - data(1) * data(4) );
    R(1,3) = 2.0 * ( data(1) * data(3) + data(2) * data(4) );
    R(2,1) = 2.0 * ( data(2) * data(3) + data(1) * data(4) );
    R(2,2) = aSq - bSq + cSq - dSq;
    R(2,3) = 2.0 * ( data(3) * data(4) - data(1) * data(2) );
    R(3,1) = 2.0 * ( data(2) * data(4) - data(1) * data(3) );
    R(3,2) = 2.0 * ( data(1) * data(2) + data(3) * data(4) );
    R(3,3) = aSq - bSq - cSq + dSq;
end

function data  = from_dcm( dcm )
    % FROM_DCM Convert DCM to quaternion
    % From https://github.com/PX4/Firmware/blob/master/src/lib/mathlib/math/Quaternion.hpp
    data = zeros(4,1);
    tr = dcm(1,1) + dcm(2,2) + dcm(3,3);
    if (tr > 0.0)
        s = sqrt(tr + 1.0);
        data(1) = s * 0.5;
        s = 0.5 / s;
        data(2) = (dcm(3,2) - dcm(2,3) ) * s;
        data(3) = (dcm(1,3) - dcm(3,1) ) * s;
        data(4) = (dcm(2,1) - dcm(1,2) ) * s;
    else
        % /* Find maximum diagonal element in dcm
        % * store index in dcm_i */
        dcm_i = 1;
        for i = 2:3 % (int i = 1; i < 3; i++)
            if ( dcm(i,i) > dcm(dcm_i,dcm_i) )
                dcm_i = i;
            end
        end
        dcm_j = rem( ( (dcm_i-1) + 1), 3) + 1;
        dcm_k = rem( ( (dcm_i-1) + 2), 3) + 1;
        s = sqrt( (dcm(dcm_i, dcm_i) - dcm(dcm_j, dcm_j) - ...
            dcm(dcm_k,dcm_k)) + 1.0 );
        data(dcm_i + 1) = s * 0.5;
        s = 0.5 / s;
        data(dcm_j + 1) = ( dcm(dcm_i,dcm_j) + dcm(dcm_j,dcm_i) ) * s;
        data(dcm_k + 1) = ( dcm(dcm_k,dcm_i) + dcm(dcm_i,dcm_k) ) * s;
        data(1) = ( dcm(dcm_k,dcm_j) - dcm(dcm_j,dcm_k) ) * s;
    end
end
